simulink model "vtg_sim_r24b_testing"  (R2024b)
settings: Solver=FixedStepAuto  StartTime=0.0  StopTime=50  FixedStep=0.05  RelTol=1e-3
InitFcn:
  | % Clear the build folder (slprj) to force a recompile of C-code
  | if exist('slprj', 'dir')
  |     rmdir('slprj', 's');
  |     fprintf('### Build cache cleared. Rebuilding C-code...\n');
  | end
settings Model: Creator=sprinkle  LastModifiedBy=Shaimaa ElBaklish
settings OptimizationCC: ReuseModelBlockBuffer=off
settings SFSimCC: SimCustomInitializer=|
  | clear mex;
  | if exist('vtg_sim_r24b_sfun.mexw64', 'file')
  |     delete('vtg_sim_r24b_sfun.mexw64');
  | end
settings RTWCC: RTWUseSimCustomCode=on  GPUComputeCapability=3.5
settings RTWCC: CustomInitializer=|
  | clear mex;
  | if exist('vtg_sim_r24b_sfun.mexw64', 'file')
  |     delete('vtg_sim_r24b_sfun.mexw64');
  | end

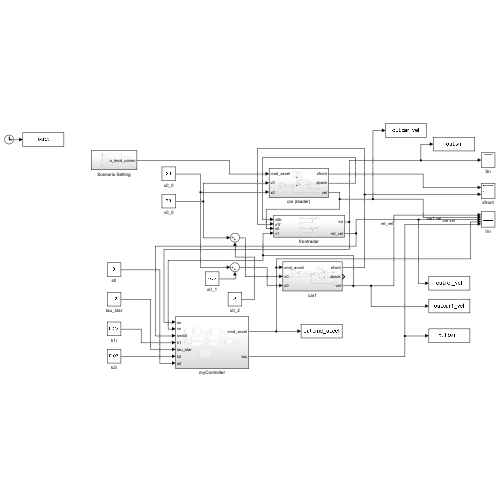
[thumbnail: Simulink's stored preview of the top-level diagram]
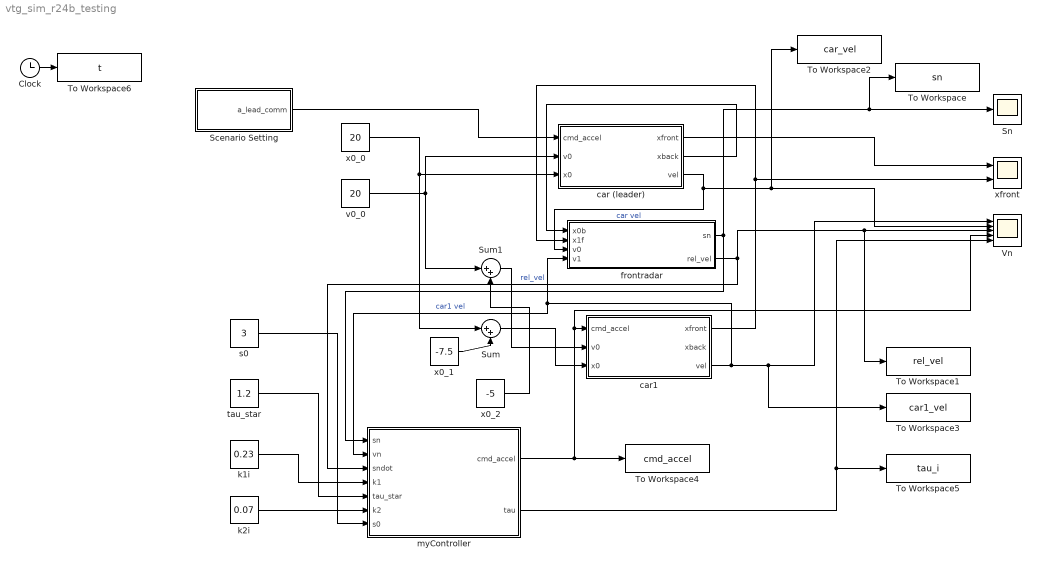
== system vtg_sim_r24b_testing ==
  Clock : Clock
  Scenario Setting : Subsystem
  Sn : Scope
  Sum : Sum  Inputs=|++
  Sum1 : Sum  Inputs=|++
  To Workspace : ToWorkspace  VariableName=sn  SampleTime=-1
  To Workspace1 : ToWorkspace  VariableName=rel_vel  SampleTime=-1
  To Workspace2 : ToWorkspace  VariableName=car_vel  SampleTime=-1
  To Workspace3 : ToWorkspace  VariableName=car1_vel  SampleTime=-1
  To Workspace4 : ToWorkspace  VariableName=cmd_accel  SampleTime=-1
  To Workspace5 : ToWorkspace  VariableName=tau_i  SampleTime=-1
  To Workspace6 : ToWorkspace  VariableName=t  SampleTime=-1
  Vn : Scope  NumInputPorts=5
  car (leader) : Subsystem
  car1 : Subsystem
  frontradar : Subsystem
  k1i : Constant  Value=0.23
  k2i : Constant  Value=0.07
  myController : Subsystem
  s0 : Constant  Value=3
  tau_star : Constant  Value=1.2
  v0_0 : Constant  Value=20
  x0_0 : Constant  Value=20
  x0_1 : Constant  Value=-7.5
  x0_2 : Constant  Value=-5
  xfront : Scope  NumInputPorts=2
  wires:
  Scenario Setting/1(a_lead_comm) -> car (leader)/1(cmd_accel)
  v0_0/1 -> car (leader)/2(v0), Sum1/1
  x0_0/1 -> Sum/1, car (leader)/3(x0)
  x0_1/1 -> Sum/2
  Sum/1 -> car1/3(x0)
  x0_2/1 -> Sum1/2
  Sum1/1 -> car1/2(v0)
  car (leader)/2(xback) -> frontradar/1(x0b)
  car1/1(xfront) -> frontradar/2(x1f), xfront/2
  car (leader)/3(vel) -> To Workspace2/1, Vn/2, frontradar/3(v0)  "car vel"
  car1/3(vel) -> To Workspace3/1, Vn/1, frontradar/4(v1), myController/2(vn)  "car1 vel"
  frontradar/2(rel_vel) -> myController/3(sndot), To Workspace1/1, Vn/3  "rel_vel"
  s0/1 -> myController/7(s0)
  tau_star/1 -> myController/5(tau_star)
  myController/1(cmd_accel) -> To Workspace4/1, Vn/4, car1/1(cmd_accel)
  k1i/1 -> myController/4(k1)
  k2i/1 -> myController/6(k2)
  myController/2(tau) -> To Workspace5/1, Vn/5
  car (leader)/1(xfront) -> xfront/1
  frontradar/1(sn) -> myController/1(sn), To Workspace/1, Sn/1
  Clock/1 -> To Workspace6/1

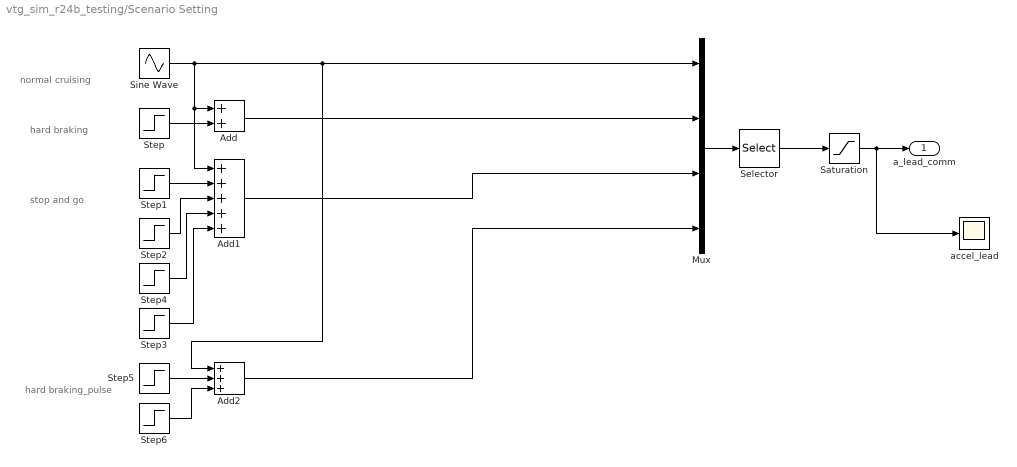
== system vtg_sim_r24b_testing/Scenario Setting ==
  note: normal cruising
  note: hard braking
  note: stop and go
  note: hard braking_pulse
  Add : Sum
  Add1 : Sum  Inputs=+++++
  Add2 : Sum  Inputs=+++
  Mux : Mux
  Saturation : Saturate  UpperLimit=1.5  LowerLimit=-3
  Selector : Selector  InputPortWidth=4  IndexOptions=Index vector (dialog)  Indices=3  OutputSizes=1
  Sine Wave : Sin  Amplitude=0.25  SampleTime=0
  Step : Step  Time=25  After=-2.5  SampleTime=0
  Step1 : Step  Time=15  After=-2  SampleTime=0
  Step2 : Step  Time=25  After=2  SampleTime=0
  Step3 : Step  Time=37  After=-2  SampleTime=0
  Step4 : Step  Time=27  After=2  SampleTime=0
  Step5 : Step  Time=25  After=-4  SampleTime=0
  Step6 : Step  Time=28  After=4  SampleTime=0
  accel_lead : Scope
  a_lead_comm : Outport
  wires:
  Sine Wave/1 -> Add/1, Add1/1, Add2/1, Mux/1
  Saturation/1 -> accel_lead/1, a_lead_comm/1
  Step/1 -> Add/2
  Add/1 -> Mux/2
  Selector/1 -> Saturation/1
  Mux/1 -> Selector/1
  Add1/1 -> Mux/3
  Step1/1 -> Add1/2
  Step2/1 -> Add1/3
  Step4/1 -> Add1/4
  Step3/1 -> Add1/5
  Add2/1 -> Mux/4
  Step5/1 -> Add2/2
  Step6/1 -> Add2/3

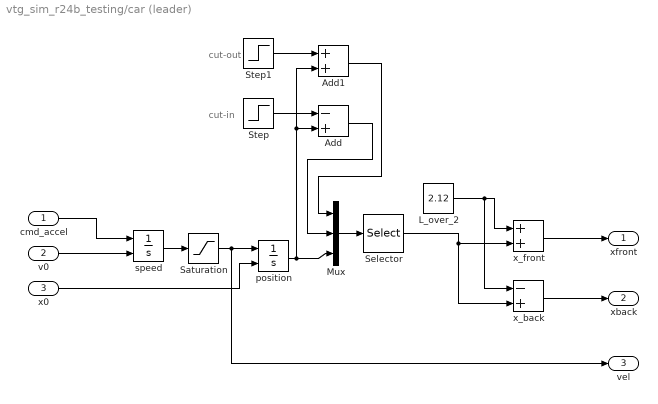
== system vtg_sim_r24b_testing/car (leader) ==
  note: cut-in
  note: cut-out
  cmd_accel : Inport
  v0 : Inport  Port=2
  x0 : Inport  Port=3
  Add : Sum  Inputs=-+
  Add1 : Sum
  L_over_2 : Constant  Value=2.12
  Mux : Mux  Inputs=3
  Saturation : Saturate  UpperLimit=inf  LowerLimit=0
  Selector : Selector  InputPortWidth=3  IndexOptions=Index vector (dialog)  Indices=3  OutputSizes=1
  Step : Step  Time=20  After=15  SampleTime=0
  Step1 : Step  Time=20  After=100  SampleTime=0
  position : Integrator  InitialConditionSource=external
  speed : Integrator  InitialConditionSource=external
  x_back : Sum  Inputs=-+
  x_front : Sum
  xfront : Outport
  xback : Outport  Port=2
  vel : Outport  Port=3
  wires:
  x_back/1 -> xback/1
  x0/1 -> position/2
  cmd_accel/1 -> speed/1
  x_front/1 -> xfront/1
  v0/1 -> speed/2
  L_over_2/1 -> x_back/1, x_front/1
  speed/1 -> Saturation/1
  Saturation/1 -> vel/1, position/1
  Selector/1 -> x_back/2, x_front/2
  Mux/1 -> Selector/1
  Step/1 -> Add/1
  Add/1 -> Mux/2
  position/1 -> Add1/2, Add/2, Mux/3
  Add1/1 -> Mux/1
  Step1/1 -> Add1/1

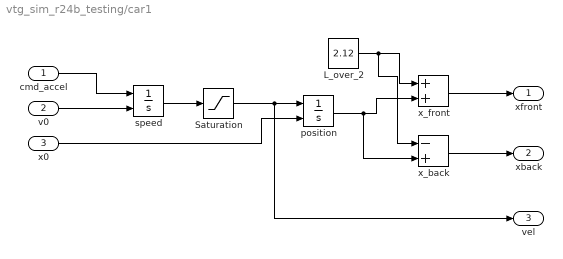
== system vtg_sim_r24b_testing/car1 ==
  cmd_accel : Inport
  v0 : Inport  Port=2
  x0 : Inport  Port=3
  L_over_2 : Constant  Value=2.12
  Saturation : Saturate  UpperLimit=inf  LowerLimit=0
  position : Integrator  InitialConditionSource=external
  speed : Integrator  InitialConditionSource=external
  x_back : Sum  Inputs=-+
  x_front : Sum
  xfront : Outport
  xback : Outport  Port=2
  vel : Outport  Port=3
  wires:
  x_back/1 -> xback/1
  x0/1 -> position/2
  cmd_accel/1 -> speed/1
  position/1 -> x_back/2, x_front/2
  x_front/1 -> xfront/1
  v0/1 -> speed/2
  L_over_2/1 -> x_back/1, x_front/1
  speed/1 -> Saturation/1
  Saturation/1 -> vel/1, position/1

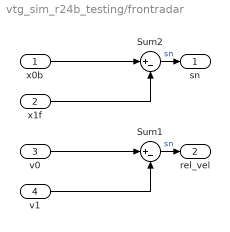
== system vtg_sim_r24b_testing/frontradar ==
  x0b : Inport
  x1f : Inport  Port=2
  v0 : Inport  Port=3
  v1 : Inport  Port=4
  Sum1 : Sum  Inputs=|+-
  Sum2 : Sum  Inputs=|+-
  sn : Outport
  rel_vel : Outport  Port=2
  wires:
  x1f/1 -> Sum2/2
  Sum2/1 -> sn/1  "sn"
  x0b/1 -> Sum2/1
  v0/1 -> Sum1/1
  Sum1/1 -> rel_vel/1  "sn"
  v1/1 -> Sum1/2

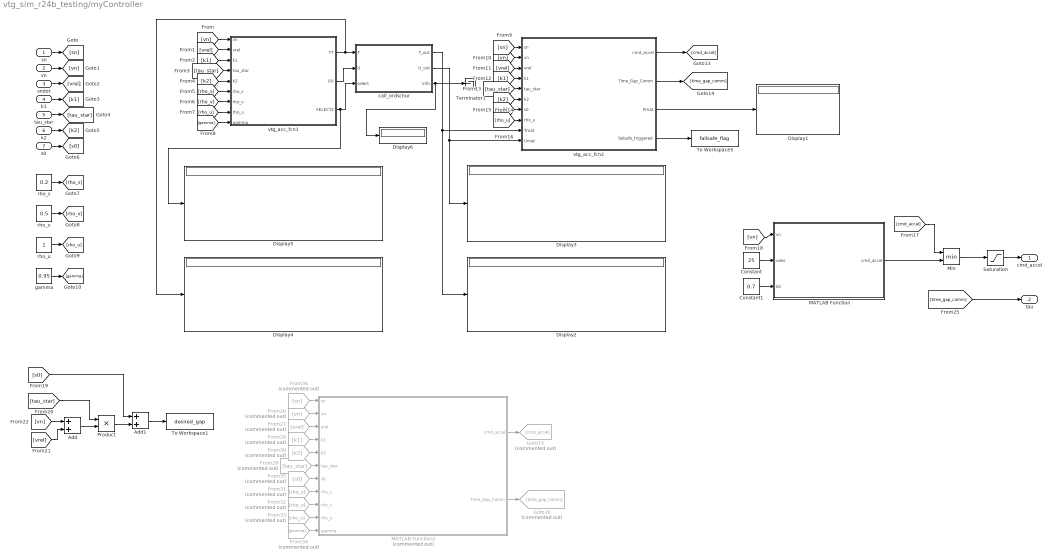
== system vtg_sim_r24b_testing/myController ==
  sn : Inport
  vn : Inport  Port=2
  sndot : Inport  Port=3
  k1 : Inport  Port=4
  tau_star : Inport  Port=5
  k2 : Inport  Port=6
  s0 : Inport  Port=7
  Add : Sum
  Add1 : Sum
  Constant : Constant  Value=25
  Constant1 : Constant  Value=0.7
  Display{1..6} (6 alike) : Display
  From26 : From  Commented=on  GotoTag=vn
  From27 : From  Commented=on  GotoTag=vrel
  From28 : From  Commented=on  GotoTag=k1
  From29 : From  Commented=on  GotoTag=tau_star
  From30 : From  Commented=on  GotoTag=k2
  From31 : From  Commented=on  GotoTag=rho_s
  From32 : From  Commented=on  GotoTag=rho_v
  From33 : From  Commented=on  GotoTag=rho_u
  From34 : From  Commented=on  GotoTag=gamma
  From35 : From  Commented=on  GotoTag=s0
  From36 : From  Commented=on  GotoTag=sn
  Goto15 : Goto  Commented=on  GotoTag=cmd_accel
  Goto16 : Goto  Commented=on  GotoTag=time_gap_comm
  MATLAB Function : MATLAB Function  TreatAsAtomicUnit=on
  MATLAB Function2 : MATLAB Function  Commented=on  TreatAsAtomicUnit=on
  Min : MinMax  Inputs=2
  Product : Product
  Saturation : Saturate  UpperLimit=1.5  LowerLimit=-3
  Terminator1 : Terminator
  To Workspace1 : ToWorkspace  VariableName=desired_gap  SampleTime=-1
  To Workspace5 : ToWorkspace  VariableName=failsafe_flag  SampleTime=-1
  call_ordschur : MATLAB Function  TreatAsAtomicUnit=on
  gamma : Constant  Value=0.95
  rho_s : Constant  Value=0.2
  rho_u : Constant
  rho_v : Constant  Value=0.5
  vtg_acc_fcn1 : MATLAB Function  TreatAsAtomicUnit=on
  vtg_acc_fcn2 : MATLAB Function  TreatAsAtomicUnit=on
  cmd_accel : Outport
  tau : Outport  Port=2
  wires:
  Saturation/1 -> cmd_accel/1
  vtg_acc_fcn1/1(TT) -> Display4/1, call_ordschur/1(T)
  vtg_acc_fcn1/2(UU) -> call_ordschur/2(U)
  vtg_acc_fcn1/3(SELECT2) -> Display5/1, call_ordschur/3(select)
  call_ordschur/1(T_out) -> vtg_acc_fcn2/9(Tmat), Display2/1
  call_ordschur/3(info) -> Terminator1/1, Display6/1
  call_ordschur/2(U_out) -> vtg_acc_fcn2/10(Umat), Display3/1
  sn/1 -> [sn]
  vn/1 -> [vn]
  sndot/1 -> [vrel]
  k1/1 -> [k1]
  tau_star/1 -> [tau_star]
  k2/1 -> [k2]
  s0/1 -> [s0]
  rho_s/1 -> [rho_s]
  rho_v/1 -> [rho_v]
  rho_u/1 -> [rho_u]
  gamma/1 -> [gamma]
  [vn] -> vtg_acc_fcn1/1(vn)
  [vrel] -> vtg_acc_fcn1/2(vrel)
  [k1] -> vtg_acc_fcn1/3(k1)
  [tau_star] -> vtg_acc_fcn1/4(tau_star)
  [k2] -> vtg_acc_fcn1/5(k2)
  [rho_s] -> vtg_acc_fcn1/6(rho_s)
  [rho_v] -> vtg_acc_fcn1/7(rho_v)
  [rho_u] -> vtg_acc_fcn1/8(rho_u)
  [gamma] -> vtg_acc_fcn1/9(gamma)
  [sn] -> vtg_acc_fcn2/1(sn)
  [vn] -> vtg_acc_fcn2/2(vn)
  [vrel] -> vtg_acc_fcn2/3(vrel)
  [k1] -> vtg_acc_fcn2/4(k1)
  [tau_star] -> vtg_acc_fcn2/5(tau_star)
  [k2] -> vtg_acc_fcn2/6(k2)
  [s0] -> vtg_acc_fcn2/7(s0)
  [rho_u] -> vtg_acc_fcn2/8(rho_u)
  vtg_acc_fcn2/3(Pmat) -> Display1/1
  Min/1 -> Saturation/1
  [time_gap_comm] -> tau/1
  vtg_acc_fcn2/1(cmd_accel) -> [cmd_accel]
  vtg_acc_fcn2/2(Time_Gap_Comm) -> [time_gap_comm]
  From34/1 -> MATLAB Function2/11(gamma)
  From31/1 -> MATLAB Function2/8(rho_s)
  From28/1 -> MATLAB Function2/4(k1)
  From26/1 -> MATLAB Function2/2(vn)
  From27/1 -> MATLAB Function2/3(vrel)
  From32/1 -> MATLAB Function2/9(rho_v)
  From30/1 -> MATLAB Function2/5(k2)
  From33/1 -> MATLAB Function2/10(rho_u)
  MATLAB Function2/1(cmd_accel) -> Goto15/1
  MATLAB Function2/2(Time_Gap_Comm) -> Goto16/1
  From35/1 -> MATLAB Function2/7(s0)
  From29/1 -> MATLAB Function2/6(tau_star)
  From36/1 -> MATLAB Function2/1(sn)
  MATLAB Function/1(cmd_accel) -> Min/2
  [cmd_accel] -> Min/1
  [vn] -> MATLAB Function/1(vn)
  Constant/1 -> MATLAB Function/2(vdes)
  Constant1/1 -> MATLAB Function/3(k0)
  vtg_acc_fcn2/4(failsafe_triggered) -> To Workspace5/1
  [vn] -> Add/1
  [vrel] -> Add/2
  Add/1 -> Product/2
  [tau_star] -> Product/1
  Product/1 -> Add1/2
  Add1/1 -> To Workspace1/1
  [s0] -> Add1/1

== matlab function vtg_sim_r24b_testing/myController/vtg_acc_fcn1 ==
  data: TT output; vn input; vrel input; k1 input; tau_star input; k2 input; UU output; rho_s input; rho_v input; rho_u input; gamma input; SELECT2 output
function [TT, UU, SELECT2] = vtg_acc_fcn1(vn, vrel, k1, tau_star, k2, rho_s, rho_v, rho_u, gamma)
Asys = [0 -1; k1 (-k1*tau_star-k2)];
Bdist = [1; k2];
Csys = [rho_s 0; 0 rho_v; 0 0];
Ru = rho_u^2;
Rmat = [-1/gamma^2 0; 0 inv(Ru)];

ve = vrel + vn;
Bctrl = [0; -k1*ve];

Bsys = [Bdist, Bctrl];
Qmat = Csys'*Csys;

% --- Replacement for icare(A, B, Q, R) -----------------------------------
Z = [Asys -(Bsys/Rmat*Bsys'); -Qmat -Asys']; % Hamiltonian
[UU, TT] = schur(Z);

% SELECT0 = real(ordeig(TT)) < 0;     % Nx1 logical
% SELECT0 = logical(SELECT0);
% % Expand pattern: [false; flag; false; flag; ...]
% N = numel(SELECT0);
% SELECT = false(2*N, 1);
% % SELECT(2:2:end) = SELECT0;
% SELECT(1:N) = SELECT0;
% 
% SELECT2 = int8(SELECT);


SELECT0 = real(ordeig(TT)) < 0;
SELECT0 = logical(SELECT0);
SELECT2 = int32(SELECT0);  % Already length 4, no expansion

end

== matlab function vtg_sim_r24b_testing/myController/MATLAB Function ==
  data: vn input; cmd_accel output; vdes input; k0 input
function cmd_accel = free_flow_fcn(vn, vdes, k0)

cmd_accel = k0 * (vdes - vn);

end

== matlab function vtg_sim_r24b_testing/myController/MATLAB Function2 ==
  settings: updateMethod=DISCRETE  sampleTime=0.05
  data: sn input; vn input; vrel input; k1 input; k2 input; tau_star input; s0 input; rho_s input; cmd_accel output; rho_v input; rho_u input; gamma input; Time_Gap_Comm output
function [cmd_accel, Time_Gap_Comm] = vtg_acc_fcn_all(sn, vn, vrel, k1, k2, tau_star, s0, rho_s, rho_v, rho_u, gamma)
% VTG_ACC_FCN  Adaptive Cruise Controller — code-generation compatible.
%
%   Replaces icare() with a closed-form bisection solver for the 2x2
%   H-infinity CARE:  A'P + PA + P*S*P + Q = 0
%
%   INPUTS
%     sn        - measured gap to leader          [m]
%     vn        - ego vehicle speed               [m/s]
%     vrel      - relative speed (leader - ego)   [m/s]
%     k1        - spacing gain                    [1/s^2]
%     tau_star  - desired time gap (ROS input)    [s],  range [0.5, 5.0]
%     k2        - speed gain                      [1/s]
%     s0        - standstill distance             [m]
%
%   OUTPUT
%     cmd_accel - commanded acceleration          [m/s^2]
%
%   ASSUMPTIONS / OPERATING RANGE
%     ve = vrel + vn (leader speed) must satisfy ve >= 10/3.6 m/s (~10 km/h).
%     Below this speed the H-inf CARE has no stabilising solution.
%     Clamp ve before calling, or use a separate stop-and-go controller.
%
%   CODE GENERATION
%     Compatible with MATLAB Coder / Simulink code generation.
%     Uses only: arithmetic, sqrt, max, a fixed-count for-loop.
%     No toolbox functions, no dynamic allocation, no while loops.
%
%   VALIDATION
%     Bisection (52 iterations) gives machine-precision agreement with
%     icare() across ve in [10,120] km/h and tau_star in [0.5,5.0] s.
%     Max element error vs icare: ~8e-16 (floating-point noise floor).
 
% ── Design constants (fixed at compile/deploy time) ───────────────────────────
rho_s  = 0.2;
rho_v  = 0.5;
rho_u  = 1.0;
gamma  = 0.95;
 
% ── Clamp ve: CARE undefined below ~7 km/h ────────────────────────────────────
% At very low leader speed, switch to a stop-and-go mode externally.
% Here we clamp to avoid a degenerate CARE; the control output will be
% physically limited downstream by the Time_Gap_Comm >= 0 saturation.
ve_min = 10.0 / 3.6;                  % 10 km/h in m/s
ve     = vrel + vn;
ve_c   = max(ve, ve_min);             % clamped leader speed for CARE only
 
% ── State errors ──────────────────────────────────────────────────────────────
s_err = sn - (s0 + tau_star * ve);    % use unclamped ve for errors
v_err = vn - ve;
 
% ── CARE coefficient scalars ──────────────────────────────────────────────────
% System matrix A = [0, -1; k1, a22]
a22 = -(k1 * tau_star + k2);
 
% Indefinite penalty matrix S = B*inv(R)*B'  (H-inf formulation)
% S = -gamma^2 * Bdist*Bdist' + rho_u^2 * Bctrl*Bctrl'
% where Bdist=[1;k2], Bctrl=[0;-k1*ve_c]
% => entries:
s11 =  gamma^2;
s12 =  gamma^2 * k2;
s22 =  gamma^2 * k2^2 - rho_u^2 * (k1 * ve_c)^2;
 
% Cost matrix Q = Csys'*Csys = diag([rho_s^2, rho_v^2])
q11 = rho_s^2;
q22 = rho_v^2;
 
% ── Closed-form CARE: solve for p12 by bisection ──────────────────────────────
%
% With P = [p11, p12; p12, p22], the CARE expands to 3 scalar equations:
%
%   eq(1,1): s11*p11^2 + 2*s12*p12*p11 + (s22*p12^2 + 2*k1*p12 + q11) = 0
%            => p11 = [-s12*p12 + sqrt(D1)] / s11           [+ root: p11>0]
%            where D1 = (s12^2 - s11*s22)*p12^2 - 2*s11*k1*p12 - s11*q11
%
%   eq(2,2): s22*p22^2 + 2*(s12*p12+a22)*p22 + (s11*p12^2 - 2*p12 + q22) = 0
%            => p22 = [-(s12*p12+a22) - sqrt(D3)] / s22     [- root: p22>0]
%            where D3 = (s12*p12+a22)^2 - s22*(s11*p12^2 - 2*p12 + q22)
%
%   eq(1,2): f(p12) = -p11 + a22*p12 + k1*p22
%                     + s11*p11*p12 + s12*(p11*p22 + p12^2) + s22*p12*p22 = 0
%
% Validated properties across ve in [10,120] km/h, tau* in [0.5,5.0] s:
%   - p12 is always in [-0.191, -0.027]  => bisect over [-0.30, -0.020]
%   - f(p12) has exactly one sign change in this interval
%   - p11 always uses + discriminant root
%   - p22 always uses - discriminant root
%
% 52 bisection iterations achieve 2^-52 ~ 2e-16 precision (machine epsilon).
 
p12_lo = -0.30;
p12_hi = -0.020;
 
for iter = 1:52                        %#ok<UNRCH>  (fixed count, code-gen safe)
    p12_mid = 0.5 * (p12_lo + p12_hi);
 
    % -- p11 and p22 at midpoint --
    D1_mid  = (s12^2 - s11*s22)*p12_mid^2 - 2*s11*k1*p12_mid - s11*q11;
    p11_mid = (-s12*p12_mid + sqrt(max(D1_mid, 0))) / s11;
 
    b_mid   = s12*p12_mid + a22;
    D3_mid  = b_mid^2 - s22*(s11*p12_mid^2 - 2*p12_mid + q22);
    p22_mid = (-b_mid - sqrt(max(D3_mid, 0))) / s22;
 
    f_mid   = -p11_mid + a22*p12_mid + k1*p22_mid ...
              + s11*p11_mid*p12_mid ...
              + s12*(p11_mid*p22_mid + p12_mid^2) ...
              + s22*p12_mid*p22_mid;
 
    % -- p11 and p22 at lo --
    D1_lo   = (s12^2 - s11*s22)*p12_lo^2 - 2*s11*k1*p12_lo - s11*q11;
    p11_lo  = (-s12*p12_lo  + sqrt(max(D1_lo,  0))) / s11;
 
    b_lo    = s12*p12_lo + a22;
    D3_lo   = b_lo^2  - s22*(s11*p12_lo^2  - 2*p12_lo  + q22);
    p22_lo  = (-b_lo  - sqrt(max(D3_lo,  0))) / s22;
 
    f_lo    = -p11_lo + a22*p12_lo + k1*p22_lo ...
              + s11*p11_lo*p12_lo ...
              + s12*(p11_lo*p22_lo + p12_lo^2) ...
              + s22*p12_lo*p22_lo;
 
    % -- Update bracket --
    if f_lo * f_mid <= 0
        p12_hi = p12_mid;
    else
        p12_lo = p12_mid;
    end
end
 
% ── Extract final P entries ───────────────────────────────────────────────────
p12 = 0.5 * (p12_lo + p12_hi);
 
D1  = (s12^2 - s11*s22)*p12^2 - 2*s11*k1*p12 - s11*q11;
p11 = (-s12*p12 + sqrt(max(D1, 0))) / s11;                    %#ok<NASGU>
 
b   = s12*p12 + a22;
D3  = b^2 - s22*(s11*p12^2 - 2*p12 + q22);
p22 = (-b - sqrt(max(D3, 0))) / s22;
 
% Note: p11 is computed above but not used in the control law (see below).
% It is retained for completeness and potential diagnostic output.
 
% ── Control law ───────────────────────────────────────────────────────────────
% ui = -(1/rho_u^2) * [0, -k1*vn] * P * [s_err; v_err]
%    = -(1/rho_u^2) * (-k1*vn) * (p12*s_err + p22*v_err)
%
% Only p12 and p22 appear here — p11 is structurally absent.
ui = -(1.0 / rho_u^2) * (-k1 * vn) * (p12 * s_err + p22 * v_err);
 
Time_Gap_Comm = max(tau_star + ui, 0);
cmd_accel     = k1 * (sn - s0 - Time_Gap_Comm * vn) + k2 * vrel;
end

== matlab function vtg_sim_r24b_testing/myController/call_ordschur ==
  data: T input; T_out output; U input; select input; U_out output; info output
function [T_out, U_out, info] = call_ordschur(T, U, select)
%#codegen
coder.cinclude('ordschur_wrapper.h');

n = size(T,1);

T_out = T;
U_out = U;

info = int32(0);

info = coder.ceval('ordschur_reorder', ...
    int32(n), ...
    coder.ref(T_out), ...
    coder.ref(U_out), ...
    coder.rref(select) );

% For Simulink
customDir = "C:\Users\ShaimaaElBaklish\Documents\GitHub\vtg_acc_real\simulink\mycfiles";
coder.updateBuildInfo('addIncludePaths', customDir);
coder.updateBuildInfo('addSourcePaths', customDir);
coder.updateBuildInfo('addSourceFiles', 'ordschur_wrapper.c');
end

== matlab function vtg_sim_r24b_testing/myController/vtg_acc_fcn2 ==
  data: sn input; cmd_accel output; vn input; vrel input; k1 input; tau_star input; k2 input; s0 input; rho_u input; Tmat input; Time_Gap_Comm output; Umat input; Pmat output; failsafe_triggered output
function [cmd_accel, Time_Gap_Comm, Pmat, failsafe_triggered] = vtg_acc_fcn2(sn, vn, vrel, k1, tau_star, k2, s0, rho_u, Tmat, Umat)
cmd_accel = 0; Time_Gap_Comm= 0; failsafe_triggered = false;
Ru = rho_u^2;

ve = vrel + vn;
s_err = sn - (s0+tau_star*ve);
v_err = vn - ve;

% --- Replacement for icare(A, B, Q, R) -----------------------------------
% diagT = diag(Tmat);
Pmat = zeros(2, 2);
[m,n] = size(Umat);
U11 = Umat(1:(m/2), 1:(n/2));
U21 = Umat((m/2+1):m, 1:(n/2));
Pmat = U21/U11;
% Pmat = 0.5*(Pmat + Pmat');
% -------------------------------------------------------------------------

ui = -inv(Ru)*([0 -k1*vn]*Pmat*[s_err; v_err]);
% if issorted(diagT)
%     Time_Gap_Comm = max(tau_star + double(ui), 0);
% else
%     % fail-safe if ordschur fails
%     Time_Gap_Comm = tau_star;
% end

% ── Check failsafe condition ───────────────────────────────────
diagT = diag(Tmat);
n     = length(diagT)/2;
failsafe_triggered = ~(all(diagT(1:n) < 0) && all(diagT(n+1:end) > 0));


Time_Gap_Comm = max(tau_star + double(ui), 0);
cmd_accel = k1*(sn-s0-Time_Gap_Comm*vn) + k2*vrel;
end
